simulink model "Electronics_II_ch1_1_10_b"  (R2013b)
settings: Solver=ode23tb  StartTime=0.0  StopTime=0.05  RelTol=1e-3
libraries: powerlib x7
settings Model: Creator=domicor  LastModifiedBy=domicor

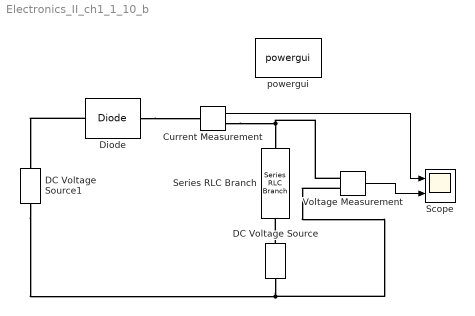
== system Electronics_II_ch1_1_10_b ==
  Current Measurement : powerlib/Measurements/Current Measurement  PhasorSimulation=off  OutputType=Complex  PSBequivalent=0
  DC Voltage Source : powerlib/Electrical Sources/DC Voltage Source  Amplitude=6  Measurements=None
  DC Voltage Source1 : powerlib/Electrical Sources/DC Voltage Source  Amplitude=9  Measurements=None
  Diode : powerlib/Power Electronics/Diode  Ron=0.00  Lon=0  Vf=0  IC=0  UseSnubber=off  Rs=500  Cs=250e-9  Measurements=off
  Scope : Scope  NumInputPorts=2
      settings: ShowLegends=on  YMin=-5~-5  YMax=5~5
  Series RLC Branch : powerlib/Elements/Series RLC Branch  LConnTagsString=__new0  RConnTagsString=__new0  BranchType=R  Resistance=3000  Inductance=1e-3  SetiL0=off  InitialCurrent=0  Capacitance=1e-6  Setx0=off  InitialVoltage=0  Measurements=None
  Voltage Measurement : powerlib/Measurements/Voltage Measurement  PhasorSimulation=off  OutputType=Complex  PSBequivalent=0
  powergui : powerlib/powergui  Priority=1  SimulationMode=Continuous  SolverType=Tustin  SampleTime=50e-6  frequency=60  SPID=on  DisableSnubberDevices=off  DisableRonSwitches=off  DisableVfSwitches=off  SwTol=0  Interpol=off  DisplayEquations=off  frequencyindice=0  Pbase=100e6  ErrMax=1e-4  Iterations=50  UnitsV=kV  UnitsW=MW  FunctionMessages=off  echomessages=off  HookPort=off  EnableUseOfTLC=off  x0status=blocks  RestoreLinks=warning  ResistiveCurrentMeasurement=off  Frange=[0:2:500]  Ylog=off  Xlog=on  ShowGrid=off  save=off  variable=ZData  ZoomFFT=off  StartTime=0.0  cycles=1  DisplayStyle=1  fundamental=60  FreqAxis=off  MaxFrequency=1000  frequencyindicesteady=1  RmsSteady=1  display=off  Ts=0  methode=off
  wires:
  Voltage Measurement/1 -> Scope/2
  Current Measurement/1 -> Scope/1
  connections:
  Voltage Measurement/LConn2 -- DC Voltage Source1/RConn1 -- DC Voltage Source/RConn1
  Voltage Measurement/LConn1 -- Current Measurement/RConn1 -- Series RLC Branch/LConn1
  Diode/RConn1 -- Current Measurement/LConn1
  DC Voltage Source/LConn1 -- Series RLC Branch/RConn1
  Diode/LConn1 -- DC Voltage Source1/LConn1
